simulink model "generator"  (R2021a)
settings: Solver=VariableStepAuto  StartTime=0.0  StopTime=tp  RelTol=1e-3
values from neighbouring files (symbols this model uses):
  np = length(points)    [Final_Project.m]
  P0 = diag([0.55 0.55 deg2rad(10)].^2)    [Final_Project.m]
  ttotal = zeros(1, np)    [Final_Project.m]
  X0 = [xx(1)-3;yy(1)-3;0.1745]    [Final_Project.m]
  Xhat0 = X0+sqrt(P0)*randn(length(X0),1)    [Final_Project.m]
  xx = [xi x1 x]    [find_path.m]
  yy = [yi y1 y]    [find_path.m]
libraries: simulink x9, robotcorelib x1
settings Model: Creator=Ferna  LastModifiedBy=Ferna

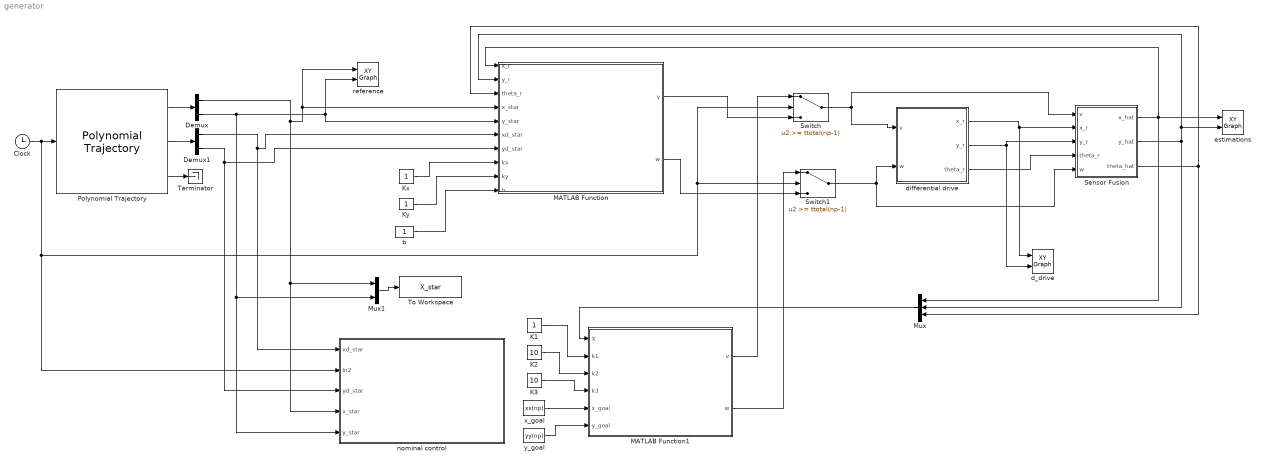
== system generator ==
  Clock : Clock
  Demux : Demux  Outputs=2
  Demux1 : Demux  Outputs=2
  K1 : Constant
  K2 : Constant  Value=10
  K3 : Constant  Value=10
  Kx : Constant
  Ky : Constant
  MATLAB Function : MATLAB Function  TreatAsAtomicUnit=on
  MATLAB Function1 : MATLAB Function  TreatAsAtomicUnit=on
  Mux : Mux  Inputs=3
  Mux1 : Mux  Inputs=2
  Polynomial Trajectory : robotcorelib/Polynomial Trajectory  WaypointSource=Internal  Waypoints=points  TimePoints=ttotal  TimeInterval=[ 1, 4 ]  Method=Quintic Polynomial  ParameterSource=Internal  VelocityBoundaryCondition=zeros(2 ,np)  AccelerationBoundaryCondition=zeros( 2, np )  SimulateUsing=Interpreted execution
  Sensor Fusion : Subsystem
  Switch : Switch  Threshold=ttotal(np-1)
  Switch1 : Switch  Threshold=ttotal(np-1)
  Terminator : Terminator
  To Workspace : ToWorkspace  VariableName=X_star  SampleTime=-1
  b : Constant
  d_drive : simulink/Sinks/XY Graph  xmin=0  xmax=100  ymin=0  ymax=100  st=-1
  differential drive : Subsystem
  estimations : simulink/Sinks/XY Graph  xmin=0  xmax=100  ymin=0  ymax=100  st=-1
  nominal control : Subsystem
  reference : simulink/Sinks/XY Graph  xmin=0  xmax=100  ymin=0  ymax=100  st=-1
  x_goal : Constant  Value=xx(np)
  y_goal : Constant  Value=yy(np)
  wires:
  Clock/1 -> nominal control/2(In2), Switch1/2, Switch/2, Polynomial Trajectory/1
  Polynomial Trajectory/3 -> Terminator/1
  Demux/1 -> nominal control/4(x_star), Mux1/1, reference/1, MATLAB Function/4(x_star)
  Demux1/1 -> nominal control/1(xd_star), MATLAB Function/6(xd_star)
  Demux1/2 -> nominal control/3(yd_star), MATLAB Function/7(yd_star)
  Kx/1 -> MATLAB Function/8(kx)
  Ky/1 -> MATLAB Function/9(ky)
  b/1 -> MATLAB Function/10(b)
  Polynomial Trajectory/2 -> Demux1/1
  Polynomial Trajectory/1 -> Demux/1
  differential drive/1(x_r) -> d_drive/1, Sensor Fusion/2(x_r)
  differential drive/2(y_r) -> d_drive/2, Sensor Fusion/3(y_r)
  Sensor Fusion/1(x_hat) -> estimations/1, MATLAB Function/1(x_r), Mux/1
  Sensor Fusion/2(y_hat) -> estimations/2, MATLAB Function/2(y_r), Mux/2
  Sensor Fusion/3(theta_hat) -> Mux/3, MATLAB Function/3(theta_r)
  differential drive/3(theta_r) -> Sensor Fusion/4(theta_r)
  Switch/1 -> differential drive/1(v), Sensor Fusion/1(v)
  Switch1/1 -> Sensor Fusion/5(w), differential drive/2(w)
  K1/1 -> MATLAB Function1/2(k1)
  K2/1 -> MATLAB Function1/3(k2)
  K3/1 -> MATLAB Function1/4(k3)
  MATLAB Function/2(w) -> Switch1/3
  MATLAB Function/1(v) -> Switch/3
  MATLAB Function1/1(v) -> Switch/1
  MATLAB Function1/2(w) -> Switch1/1
  x_goal/1 -> MATLAB Function1/5(x_goal)
  y_goal/1 -> MATLAB Function1/6(y_goal)
  Mux1/1 -> To Workspace/1
  Demux/2 -> nominal control/5(y_star), Mux1/2, MATLAB Function/5(y_star), reference/2
  Mux/1 -> MATLAB Function1/1(X)

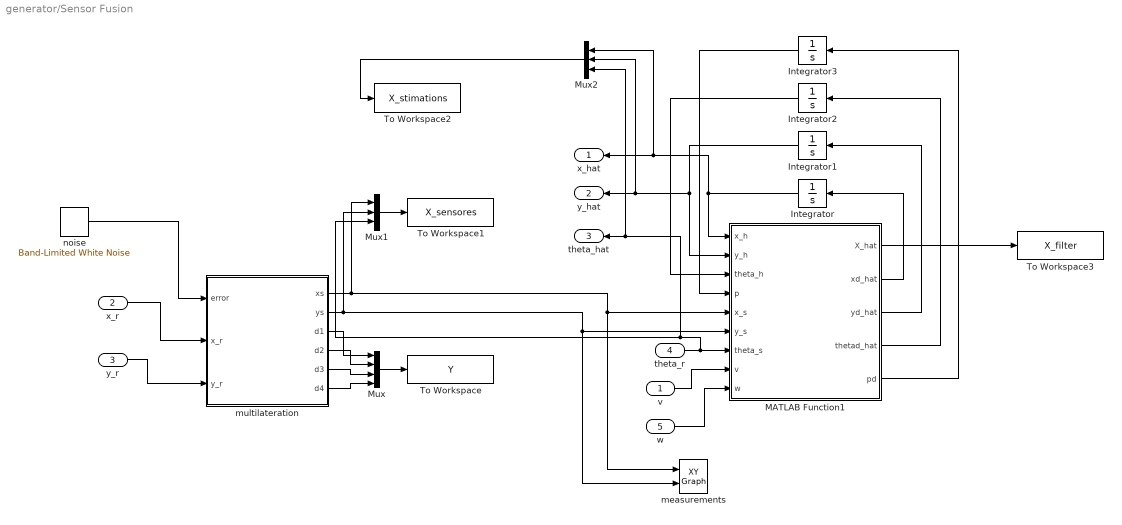
== system generator/Sensor Fusion ==
  v : Inport
  x_r : Inport  Port=2
  y_r : Inport  Port=3
  theta_r : Inport  Port=4
  w : Inport  Port=5
  Integrator : Integrator  InitialCondition=Xhat0(1)
  Integrator1 : Integrator  InitialCondition=Xhat0(2)
  Integrator2 : Integrator  InitialCondition=Xhat0(3)
  Integrator3 : Integrator  InitialCondition=P0
  MATLAB Function1 : MATLAB Function  TreatAsAtomicUnit=on
  Mux : Mux
  Mux1 : Mux  Inputs=3
  Mux2 : Mux  Inputs=3
  To Workspace : ToWorkspace  VariableName=Y  SampleTime=-1
  To Workspace1 : ToWorkspace  VariableName=X_sensores  SampleTime=-1
  To Workspace2 : ToWorkspace  VariableName=X_stimations  SampleTime=-1
  To Workspace3 : ToWorkspace  VariableName=X_filter  SampleTime=-1
  measurements : simulink/Sinks/XY Graph  xmin=0  xmax=100  ymin=0  ymax=100  st=-1
  multilateration : MATLAB Function  TreatAsAtomicUnit=on
  noise : simulink/Sources/Band-Limited White Noise  Cov=[0.01]  Ts=0.08  seed=[52523]
  x_hat : Outport
  y_hat : Outport  Port=2
  theta_hat : Outport  Port=3
  wires:
  MATLAB Function1/4(thetad_hat) -> Integrator2/1
  Integrator/1 -> MATLAB Function1/1(x_h), Mux2/1, x_hat/1
  Integrator3/1 -> MATLAB Function1/4(p)
  MATLAB Function1/2(xd_hat) -> Integrator/1
  v/1 -> MATLAB Function1/8(v)
  Integrator2/1 -> MATLAB Function1/3(theta_h)
  MATLAB Function1/3(yd_hat) -> Integrator1/1
  multilateration/2(ys) -> Mux1/2, measurements/2, MATLAB Function1/6(y_s)
  multilateration/1(xs) -> Mux1/1, measurements/1, MATLAB Function1/5(x_s)
  Integrator1/1 -> Mux2/2, y_hat/1, MATLAB Function1/2(y_h)
  MATLAB Function1/5(pd) -> Integrator3/1
  y_r/1 -> multilateration/3(y_r)
  w/1 -> MATLAB Function1/9(w)
  x_r/1 -> multilateration/2(x_r)
  theta_r/1 -> Mux2/3, theta_hat/1, Mux1/3, MATLAB Function1/7(theta_s)
  Mux/1 -> To Workspace/1
  multilateration/3(d1) -> Mux/1
  multilateration/4(d2) -> Mux/2
  multilateration/5(d3) -> Mux/3
  multilateration/6(d4) -> Mux/4
  Mux1/1 -> To Workspace1/1
  noise/1 -> multilateration/1(error)
  Mux2/1 -> To Workspace2/1
  MATLAB Function1/1(X_hat) -> To Workspace3/1

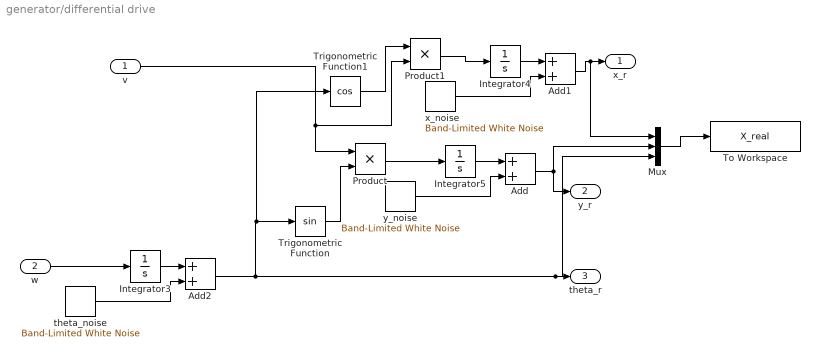
== system generator/differential drive ==
  v : Inport
  w : Inport  Port=2
  Add : Sum
  Add1 : Sum
  Add2 : Sum
  Integrator3 : Integrator  InitialCondition=X0(3)
  Integrator4 : Integrator  InitialCondition=X0(1)
  Integrator5 : Integrator  InitialCondition=X0(2)
  Mux : Mux  Inputs=3
  Product : Product
  Product1 : Product
  To Workspace : ToWorkspace  VariableName=X_real  SampleTime=-1
  Trigonometric Function : Trigonometry
  Trigonometric Function1 : Trigonometry  Operator=cos
  theta_noise : simulink/Sources/Band-Limited White Noise  Cov=[0.001]  Ts=0.08  seed=[12634]
  x_noise : simulink/Sources/Band-Limited White Noise  Cov=[0.005]  Ts=0.08  seed=[76523]
  y_noise : simulink/Sources/Band-Limited White Noise  Cov=[0.005]  Ts=0.08  seed=[29385]
  x_r : Outport
  y_r : Outport  Port=2
  theta_r : Outport  Port=3
  wires:
  v/1 -> Product/1, Product1/2
  Product1/1 -> Integrator4/1
  w/1 -> Integrator3/1
  Trigonometric Function/1 -> Product/2
  Trigonometric Function1/1 -> Product1/1
  Product/1 -> Integrator5/1
  y_noise/1 -> Add/2
  Integrator5/1 -> Add/1
  Add/1 -> y_r/1, Mux/2
  x_noise/1 -> Add1/2
  Integrator4/1 -> Add1/1
  Add1/1 -> Mux/1, x_r/1
  theta_noise/1 -> Add2/2
  Integrator3/1 -> Add2/1
  Add2/1 -> Mux/3, theta_r/1, Trigonometric Function1/1, Trigonometric Function/1
  Mux/1 -> To Workspace/1

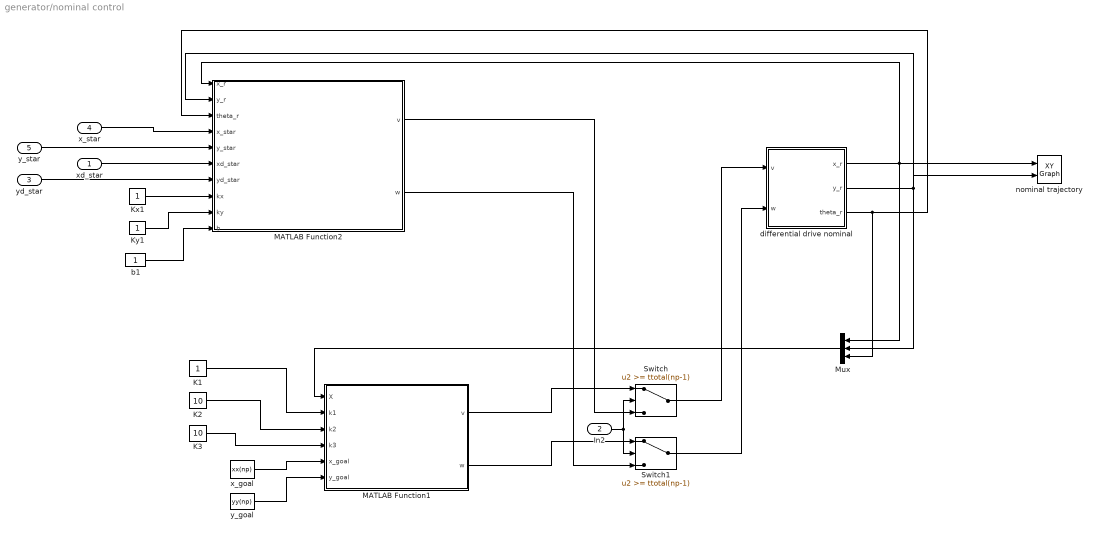
== system generator/nominal control ==
  xd_star : Inport
  In2 : Inport  Port=2
  yd_star : Inport  Port=3
  x_star : Inport  Port=4
  y_star : Inport  Port=5
  " nominal trajectory" : simulink/Sinks/XY Graph  xmin=0  xmax=100  ymin=0  ymax=100  st=-1
  K1 : Constant
  K2 : Constant  Value=10
  K3 : Constant  Value=10
  Kx1 : Constant
  Ky1 : Constant
  MATLAB Function1 : MATLAB Function  TreatAsAtomicUnit=on
  MATLAB Function2 : MATLAB Function  TreatAsAtomicUnit=on
  Mux : Mux  Inputs=3
  Switch : Switch  Threshold=ttotal(np-1)
  Switch1 : Switch  Threshold=ttotal(np-1)
  b1 : Constant
  differential drive nominal : Subsystem
  x_goal : Constant  Value=xx(np)
  y_goal : Constant  Value=yy(np)
  wires:
  differential drive nominal/1(x_r) -> Mux/1, " nominal trajectory"/1, MATLAB Function2/1(x_r)
  b1/1 -> MATLAB Function2/10(b)
  yd_star/1 -> MATLAB Function2/7(yd_star)
  Ky1/1 -> MATLAB Function2/9(ky)
  xd_star/1 -> MATLAB Function2/6(xd_star)
  Kx1/1 -> MATLAB Function2/8(kx)
  differential drive nominal/2(y_r) -> MATLAB Function2/2(y_r), Mux/2, " nominal trajectory"/2
  differential drive nominal/3(theta_r) -> Mux/3, MATLAB Function2/3(theta_r)
  y_star/1 -> MATLAB Function2/5(y_star)
  x_star/1 -> MATLAB Function2/4(x_star)
  K2/1 -> MATLAB Function1/3(k2)
  y_goal/1 -> MATLAB Function1/6(y_goal)
  K1/1 -> MATLAB Function1/2(k1)
  x_goal/1 -> MATLAB Function1/5(x_goal)
  K3/1 -> MATLAB Function1/4(k3)
  Mux/1 -> MATLAB Function1/1(X)
  MATLAB Function1/1(v) -> Switch/1
  MATLAB Function1/2(w) -> Switch1/1
  Switch/1 -> differential drive nominal/1(v)
  Switch1/1 -> differential drive nominal/2(w)
  MATLAB Function2/1(v) -> Switch/3
  MATLAB Function2/2(w) -> Switch1/3
  In2/1 -> Switch/2, Switch1/2

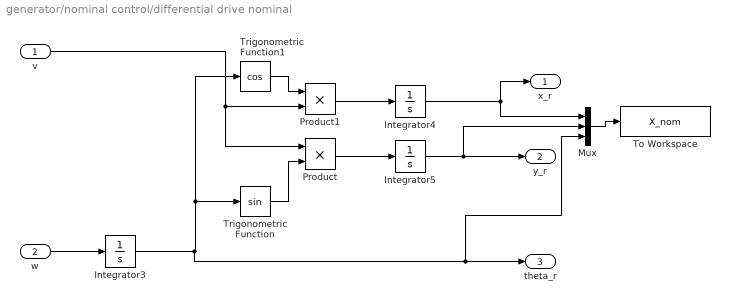
== system generator/nominal control/differential drive nominal ==
  v : Inport
  w : Inport  Port=2
  Integrator3 : Integrator  InitialCondition=X0(3)
  Integrator4 : Integrator  InitialCondition=X0(1)
  Integrator5 : Integrator  InitialCondition=X0(2)
  Mux : Mux  Inputs=3
  Product : Product
  Product1 : Product
  To Workspace : ToWorkspace  VariableName=X_nom  SampleTime=-1
  Trigonometric Function : Trigonometry
  Trigonometric Function1 : Trigonometry  Operator=cos
  x_r : Outport
  y_r : Outport  Port=2
  theta_r : Outport  Port=3
  wires:
  Mux/1 -> To Workspace/1
  Integrator3/1 -> theta_r/1, Mux/3, Trigonometric Function/1, Trigonometric Function1/1
  Integrator4/1 -> x_r/1, Mux/1
  Integrator5/1 -> Mux/2, y_r/1
  Product/1 -> Integrator5/1
  Trigonometric Function1/1 -> Product1/1
  Trigonometric Function/1 -> Product/2
  w/1 -> Integrator3/1
  Product1/1 -> Integrator4/1
  v/1 -> Product/1, Product1/2

== matlab function generator/nominal control/MATLAB Function1 ==
  data: X input; v output; k1 input; k2 input; w output; k3 input; x_goal input; y_goal input
function [v,w] = posture_reg(X,k1,k2,k3,x_goal,y_goal)
x=X(1);
y=X(2);
theta=X(3);

x_star=x_goal;
y_star=y_goal;
theta_star=pi;

ex=x_star-x;
ey=y_star-y;
etheta=delta_angle(theta_star,theta);

rho=norm([ex;ey]);
gamma=delta_angle(atan2(ey,ex),theta);
delta=delta_angle(gamma,etheta);

v=k1*rho*cos(gamma);
w=k2*gamma+k1*(sin(gamma)*cos(gamma)/gamma)*(gamma+k3*delta);
end

== matlab function generator/Sensor Fusion/multilateration ==
  settings: updateMethod=DISCRETE
  data: error input; x_r input; xs output; y_r input; ys output; d1 output; d2 output; d3 output; d4 output
function [xs,ys,d1,d2,d3,d4] = multilateration(error, x_r,y_r)
rng(3000);
N=4;% num beacons
% Rmin=1; %radio max beacon
% Rmax=70; %radio min beacon
xReal=[x_r;y_r];
%V1=normrnd(0,2.5,1,N)';
sigma_0=1;
f=@(theta,beacons)(sqrt((beacons(:,1)-theta(1)).^2+(beacons(:,2)-theta(2)).^2));
beacons=[24 25;
         24 73;
         67 75;
         70 30];
d=f(xReal,beacons);
dhat=d+error*randn(4,1);
d1=dhat(1);
d2=dhat(2);
d3=dhat(3);
d4=dhat(4);
theta0=xReal+sigma_0*randn(2,1);
%% tecnica 1
J=zeros(N,2);
for k=1:N
    xc=beacons(k,1);
    yc=beacons(k,2);
    dc=norm(beacons(k,:)-theta0(:)');
    Jx=(theta0(1)-xc)/dc;
    Jy=(theta0(2)-yc)/dc;
    J(k,:)=[Jx Jy];
end
theta_hat1=theta0+pinv(J)*(dhat-f(theta0,beacons));
xs=theta_hat1(1);
ys=theta_hat1(2);

== matlab function generator/MATLAB Function ==
  data: x_r input; v output; y_r input; theta_r input; x_star input; y_star input; xd_star input; yd_star input; kx input; ky input; b input; w output
function [v,w] = control_IO_L(x_r,y_r,theta_r,x_star,y_star,xd_star,yd_star,kx,ky,b)
x=x_r;
y=y_r;
theta=theta_r;

xB=x+b*cos(theta);
yB=y+b*sin(theta);

xstar=x_star;
ystar=y_star;

xBdotstar=xd_star;
yBdotstar=yd_star;


Tinv=[
     cos(theta)   sin(theta);
    -sin(theta)/b cos(theta)/b
    ];
ux=xBdotstar+kx*(xstar-xB);
uy=yBdotstar+ky*(ystar-yB);

vw=Tinv*[ux;uy];
v=vw(1);
w=vw(2);
% xdot=v*cos(theta);
% ydot=v*sin(theta);
% thetadot=w;

== matlab function generator/Sensor Fusion/MATLAB Function1 ==
  data: X_hat output; x_h input; y_h input; theta_h input; p input; x_s input; xd_hat output; y_s input; theta_s input; v input; w input; yd_hat output; thetad_hat output; pd output
function [X_hat,xd_hat,yd_hat,thetad_hat,pd] = EKF_CT(x_h,y_h,theta_h,p,x_s,y_s,theta_s, v,w)
% sensor values
x_m=x_s; 
y_m=y_s;
theta_m=theta_s;
%______Inputs_________%
u1=v;
u2=w;
%____covariances____%
v1=10*eye(3);% in the model
v2=0.1*eye(3);% in the measurements
pkk_1=p;
C=[1 0 0;
    0 1 0;
    0 0 1];
%measurements 
ym=[x_m;y_m;theta_m];
% kalman gain
L=pkk_1*C*inv(C*pkk_1*C+v2);
%stimate the output
Yhatkk_1=C*[x_h;y_h;theta_h];
%innotaviton
ee=ym-Yhatkk_1;
% states filteres xhat(k/k)
Xhatkk=[x_h;y_h;theta_h]+L*ee;
X_hat=Xhatkk;
% covariance filtered
Pkk=pkk_1-L*C*pkk_1;
% presiction of states
xd_hat=u1*cos(Xhatkk(3));
yd_hat=u1*sin(Xhatkk(3));
thetad_hat=u2;
% linearization of matrix A around the stimation
A=[0, 0, -u1*sin(theta_h);
   0, 0,  u1*cos(theta_h);
   0, 0,      0];
% prediction of the covariance 
pd=A*Pkk*A'+v1;

== matlab function generator/MATLAB Function1 ==
  data: X input; v output; k1 input; k2 input; w output; k3 input; x_goal input; y_goal input
function [v,w] = posture_reg(X,k1,k2,k3,x_goal,y_goal)
x=X(1);
y=X(2);
theta=X(3);

x_star=x_goal;
y_star=y_goal;
theta_star=pi;

ex=x_star-x;
ey=y_star-y;
etheta=delta_angle(theta_star,theta);

rho=norm([ex;ey]);
gamma=delta_angle(atan2(ey,ex),theta);
delta=delta_angle(gamma,etheta);

v=k1*rho*cos(gamma);
w=k2*gamma+k1*(sin(gamma)*cos(gamma)/gamma)*(gamma+k3*delta);
end

== matlab function generator/nominal control/MATLAB Function2 ==
  data: x_r input; v output; y_r input; theta_r input; x_star input; y_star input; xd_star input; yd_star input; kx input; ky input; b input; w output
function [v,w] = control_IO_L(x_r,y_r,theta_r,x_star,y_star,xd_star,yd_star,kx,ky,b)
x=x_r;
y=y_r;
theta=theta_r;

xB=x+b*cos(theta);
yB=y+b*sin(theta);

xstar=x_star;
ystar=y_star;

xBdotstar=xd_star;
yBdotstar=yd_star;


Tinv=[
     cos(theta)   sin(theta);
    -sin(theta)/b cos(theta)/b
    ];
ux=xBdotstar+kx*(xstar-xB);
uy=yBdotstar+ky*(ystar-yB);

vw=Tinv*[ux;uy];
v=vw(1);
w=vw(2);
% xdot=v*cos(theta);
% ydot=v*sin(theta);
% thetadot=w;
